simulink model "coil_ironcore_b"  (R2024a)
settings: Solver=VariableStepAuto  StartTime=0.0  StopTime=te  MaxStep=te/500  RelTol=1e-3
values from neighbouring files (symbols this model uses):
  R = 10    [sim21_solution.m]
  U = 230*sqrt(2)    [sim21_solution.m]
  w = [0.5 1 2]    [sim21_solution.m]
undefined symbols (not defined in the file or in its folder): A, B, H, l, N
settings Model: Creator=ocean  LastModifiedBy=ocean

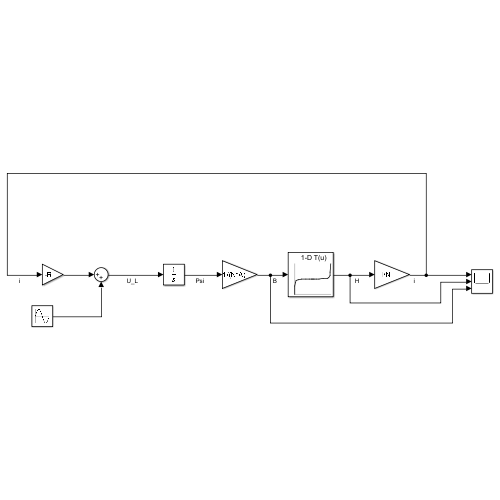
[thumbnail: Simulink's stored preview of the top-level diagram]
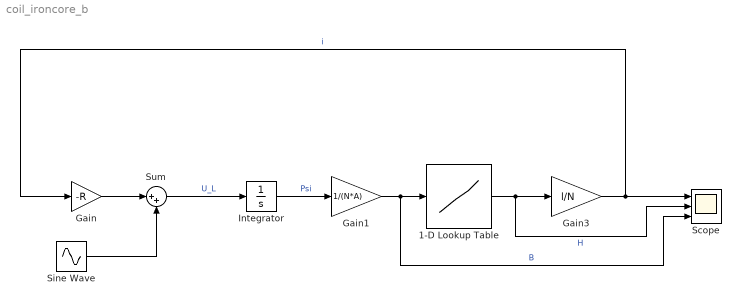
== system coil_ironcore_b ==
  1-D Lookup Table : Lookup_n-D  NumberOfTableDimensions=1  BreakpointsForDimension1=B  Table=H  InternalRulePriority=Speed  RndMeth=Simplest
  Gain : Gain  Gain=-R
  Gain1 : Gain  Gain=1/(N*A)
  Gain3 : Gain  Gain=l/N
  Integrator : Integrator
  Scope : Scope  NumInputPorts=3
  Sine Wave : Sin  Amplitude=U  Frequency=w  SampleTime=0
  Sum : Sum  Inputs=|++
  wires:
  Sine Wave/1 -> Sum/2
  Gain/1 -> Sum/1
  Sum/1 -> Integrator/1  "U_L"
  Integrator/1 -> Gain1/1  "Psi"
  Gain1/1 -> Scope/3, 1-D Lookup Table/1  "B"
  1-D Lookup Table/1 -> Scope/2, Gain3/1  "H"
  Gain3/1 -> Gain/1, Scope/1  "i"
